simulink model "sm_car"  (R2022a)
settings: Solver=ode23t  StartTime=0.0  StopTime=200  MaxStep=0.4  RelTol=1e-3  AbsTol=1e-3  EnableMultiTasking=on
PreLoadFcn:
  | disp('Loading default data for 2-axle vehicle and 1-axle trailer.')
  | if verLessThan('matlab', '9.11')
  |     load Vehicle_139
  |     Vehicle = Vehicle_139;
  |     load Trailer_01
  |     Trailer = Trailer_01;
  | else
  |     load Vehicle_189
  |     Vehicle = Vehicle_189;
  |     load Trailer_07
  |     Trailer = Trailer_07;
  | end
  | 
  | disp('Turning off MFEval warnings...')
  | disp('Solver:CoeffChecks:Eyk -- OFF')
  | disp('Solver:Limits:Exceeded -- OFF')
  | disp('Solver:CoeffChecks:Et -- OFF')
  | disp('Solver:CoeffChecks:Exa -- OFF')
  | 
  | warning('off','Solver:CoeffChecks:Eyk')
  | warning('off','Solver:Limits:Exceeded')
  | warning('off','Solver:CoeffChecks:Et')
  | warning('off','Solver:CoeffChecks:Exa')
  | %warning('off','Solver:Radius:NegativeRho')
  | 
  | % Due to usability issue in Repeating Sequence block
  | warning('off','Simulink:Masking:Invalid');
  | 
  | % Eliminate unnecessary warnings in inactive variants
  | % Warnings generated only if you click through inactive variant
  | warning('off','MATLAB:nonExistentField');
  | warning('off','Simulink:Parameters:BlkParamUndefined');
PostLoadFcn:
  | disp('Disabling trailer by default.')
  | set_param([bdroot '/Vehicle'],'popup_trailer','Off')
  | warning('off','sm:sli:setup:compile:LocalSolverNotSupported')
  | sm_car_config_maneuver(bdroot,'WOT Braking');
  | sm_car_config_vehicle(bdroot);
  | sm_car_config_logging(bdroot);
InitFcn:
  | sm_car_config_camera;
  | Vehicle = sm_car_vehcfg_checkConfig(Vehicle);
  | sm_car_check_tire_model(bdroot);
  | addpath('C:\MasterThesis_CEVT\code\casadi-windows-matlabR2016a-v3.5.5')
  | addpath('C:\MasterThesis_CEVT\code')
  | addpath('C:\MasterThesis_CEVT\code\python scripts')
StartFcn:
  | tic;
StopFcn:
  | Elapsed_Sim_Time = toc;
  | % disp(['Elapsed Sim Time = ' num2str(Elapsed_Sim_Time)]);
  | % Run script that exports relevant simulation data to json
  | simToJson
undefined symbols (not defined in the file or in its folder): Control, Driver, Maneuver
libraries: sm_car_lib x22, simulink x17, sm_lib x3, Vehicle_Visualization x3, Driver_Long_Lat_Stanley x2, Maneuver_Get_Pose x2, Camera_Frame_Definitions x1, Control_FuelCell1Motor x1, slpidlib x1, Driver_Drive_Cycle x1, Driver_Gamepad_Xbox x1, Driver_Open_Loop x1
(part 3 of 3)

== system sm_car/Vehicle/Vehicle Constraint/No Yaw ==
  Cartesian Joint : sm_lib/Joints/Cartesian Joint  JointMode=Normal  SenseConstraintForce=off  SenseConstraintForceX=off  SenseConstraintForceY=off  SenseConstraintForceZ=off  SenseConstraintTorque=off  SenseConstraintTorqueX=off  SenseConstraintTorqueY=off  SenseConstraintTorqueZ=off  SenseTotalForce=off  SenseTotalForceX=off  SenseTotalForceY=off  SenseTotalForceZ=off  SenseTotalTorque=off  SenseTotalTorqueX=off  SenseTotalTorqueY=off  SenseTotalTorqueZ=off  CompositeWrenchDir=FollowerOnBase  CompositeWrenchFrame=BaseFrame  PxEquilibriumPosition=0  PxEquilibriumPositionUnits=m  PxSpringStiffness=0  PxSpringStiffnessUnits=N/m  PxDampingCoefficient=0  PxDampingCoefficientUnits=N/(m/s)  PxTorqueActuationMode=NoTorque  PxMotionActuationMode=ComputedMotion  PxSensePosition=off  PxSenseVelocity=off  PxSenseAcceleration=off  PxSenseTorqueForce=off  PxSenseLowerLimitTorqueForce=off  PxSenseUpperLimitTorqueForce=off  PxLowerLimitSpecify=off  PxLowerLimitBound=-1  PxLowerLimitBoundUnits=m  PxLowerLimitStiffness=1e6  PxLowerLimitStiffnessUnits=N/m  PxLowerLimitDamping=1e3  PxLowerLimitDampingUnits=N/(m/s)  PxLowerLimitTransitionRegionWidth=1e-4  PxLowerLimitTransitionRegionWidthUnits=m  PxUpperLimitSpecify=off  PxUpperLimitBound=1  PxUpperLimitBoundUnits=m  PxUpperLimitStiffness=1e6  PxUpperLimitStiffnessUnits=N/m  PxUpperLimitDamping=1e3  PxUpperLimitDampingUnits=N/(m/s)  PxUpperLimitTransitionRegionWidth=1e-4  PxUpperLimitTransitionRegionWidthUnits=m  PxPositionTargetSpecify=off  PxPositionTargetPriority=High  PxPositionTargetValue=0  PxPositionTargetValueUnits=m  PxVelocityTargetSpecify=off  PxVelocityTargetPriority=High  PxVelocityTargetValue=0  PxVelocityTargetValueUnits=m/s  PyEquilibriumPosition=0  PyEquilibriumPositionUnits=m  PySpringStiffness=0  PySpringStiffnessUnits=N/m  PyDampingCoefficient=0  PyDampingCoefficientUnits=N/(m/s)  PyTorqueActuationMode=NoTorque  PyMotionActuationMode=ComputedMotion  PySensePosition=off  PySenseVelocity=off  PySenseAcceleration=off  PySenseTorqueForce=off  PySenseLowerLimitTorqueForce=off  PySenseUpperLimitTorqueForce=off  PyLowerLimitSpecify=off  PyLowerLimitBound=-1  PyLowerLimitBoundUnits=m  PyLowerLimitStiffness=1e6  PyLowerLimitStiffnessUnits=N/m  PyLowerLimitDamping=1e3  PyLowerLimitDampingUnits=N/(m/s)  PyLowerLimitTransitionRegionWidth=1e-4  PyLowerLimitTransitionRegionWidthUnits=m  PyUpperLimitSpecify=off  PyUpperLimitBound=1  PyUpperLimitBoundUnits=m  PyUpperLimitStiffness=1e6  PyUpperLimitStiffnessUnits=N/m  PyUpperLimitDamping=1e3  PyUpperLimitDampingUnits=N/(m/s)  PyUpperLimitTransitionRegionWidth=1e-4  PyUpperLimitTransitionRegionWidthUnits=m  PyPositionTargetSpecify=off  PyPositionTargetPriority=High  PyPositionTargetValue=0  PyPositionTargetValueUnits=m  PyVelocityTargetSpecify=off  PyVelocityTargetPriority=High  PyVelocityTargetValue=0  PyVelocityTargetValueUnits=m/s  PzEquilibriumPosition=0  PzEquilibriumPositionUnits=m  PzSpringStiffness=0  PzSpringStiffnessUnits=N/m  PzDampingCoefficient=0  PzDampingCoefficientUnits=N/(m/s)  PzTorqueActuationMode=NoTorque  PzMotionActuationMode=ComputedMotion  PzSensePosition=off  PzSenseVelocity=off  PzSenseAcceleration=off  PzSenseTorqueForce=off  PzSenseLowerLimitTorqueForce=off  PzSenseUpperLimitTorqueForce=off  PzLowerLimitSpecify=off  PzLowerLimitBound=-1  PzLowerLimitBoundUnits=m  PzLowerLimitStiffness=1e6  PzLowerLimitStiffnessUnits=N/m  PzLowerLimitDamping=1e3  PzLowerLimitDampingUnits=N/(m/s)  PzLowerLimitTransitionRegionWidth=1e-4  PzLowerLimitTransitionRegionWidthUnits=m  PzUpperLimitSpecify=off  PzUpperLimitBound=1  PzUpperLimitBoundUnits=m  PzUpperLimitStiffness=1e6  PzUpperLimitStiffnessUnits=N/m  PzUpperLimitDamping=1e3  PzUpperLimitDampingUnits=N/(m/s)  PzUpperLimitTransitionRegionWidth=1e-4  PzUpperLimitTransitionRegionWidthUnits=m  PzPositionTargetSpecify=off  PzPositionTargetPriority=High  PzPositionTargetValue=0  PzPositionTargetValueUnits=m  PzVelocityTargetSpecify=off  PzVelocityTargetPriority=High  PzVelocityTargetValue=0  PzVelocityTargetValueUnits=m/s
  Universal Joint : sm_lib/Joints/Universal Joint  JointMode=Normal  SenseConstraintForce=off  SenseConstraintForceX=off  SenseConstraintForceY=off  SenseConstraintForceZ=off  SenseConstraintTorque=off  SenseConstraintTorqueX=off  SenseConstraintTorqueY=off  SenseConstraintTorqueZ=off  SenseTotalForce=off  SenseTotalForceX=off  SenseTotalForceY=off  SenseTotalForceZ=off  SenseTotalTorque=off  SenseTotalTorqueX=off  SenseTotalTorqueY=off  SenseTotalTorqueZ=off  CompositeWrenchDir=FollowerOnBase  CompositeWrenchFrame=BaseFrame  RxEquilibriumPosition=0  RxEquilibriumPositionUnits=deg  RxSpringStiffness=0  RxSpringStiffnessUnits=N*m/deg  RxDampingCoefficient=0  RxDampingCoefficientUnits=N*m/(deg/s)  RxTorqueActuationMode=NoTorque  RxMotionActuationMode=ComputedMotion  RxSensePosition=off  RxSenseVelocity=off  RxSenseAcceleration=off  RxSenseTorqueForce=off  RxSenseLowerLimitTorqueForce=off  RxSenseUpperLimitTorqueForce=off  RxLowerLimitSpecify=off  RxLowerLimitBound=-90  RxLowerLimitBoundUnits=deg  RxLowerLimitStiffness=1e4  RxLowerLimitStiffnessUnits=N*m/deg  RxLowerLimitDamping=10  RxLowerLimitDampingUnits=N*m/(deg/s)  RxLowerLimitTransitionRegionWidth=0.1  RxLowerLimitTransitionRegionWidthUnits=deg  RxUpperLimitSpecify=off  RxUpperLimitBound=90  RxUpperLimitBoundUnits=deg  RxUpperLimitStiffness=1e4  RxUpperLimitStiffnessUnits=N*m/deg  RxUpperLimitDamping=10  RxUpperLimitDampingUnits=N*m/(deg/s)  RxUpperLimitTransitionRegionWidth=0.1  RxUpperLimitTransitionRegionWidthUnits=deg  RxPositionTargetSpecify=off  RxPositionTargetPriority=High  RxPositionTargetValue=0  RxPositionTargetValueUnits=deg  RxVelocityTargetSpecify=off  RxVelocityTargetPriority=High  RxVelocityTargetValue=0  RxVelocityTargetValueUnits=deg/s  RyEquilibriumPosition=0  RyEquilibriumPositionUnits=deg  RySpringStiffness=0  RySpringStiffnessUnits=N*m/deg  RyDampingCoefficient=0  RyDampingCoefficientUnits=N*m/(deg/s)  RyTorqueActuationMode=NoTorque  RyMotionActuationMode=ComputedMotion  RySensePosition=off  RySenseVelocity=off  RySenseAcceleration=off  RySenseTorqueForce=off  RySenseLowerLimitTorqueForce=off  RySenseUpperLimitTorqueForce=off  RyLowerLimitSpecify=off  RyLowerLimitBound=-90  RyLowerLimitBoundUnits=deg  RyLowerLimitStiffness=1e4  RyLowerLimitStiffnessUnits=N*m/deg  RyLowerLimitDamping=10  RyLowerLimitDampingUnits=N*m/(deg/s)  RyLowerLimitTransitionRegionWidth=0.1  RyLowerLimitTransitionRegionWidthUnits=deg  RyUpperLimitSpecify=off  RyUpperLimitBound=90  RyUpperLimitBoundUnits=deg  RyUpperLimitStiffness=1e4  RyUpperLimitStiffnessUnits=N*m/deg  RyUpperLimitDamping=10  RyUpperLimitDampingUnits=N*m/(deg/s)  RyUpperLimitTransitionRegionWidth=0.1  RyUpperLimitTransitionRegionWidthUnits=deg  RyPositionTargetSpecify=off  RyPositionTargetPriority=High  RyPositionTargetValue=0  RyPositionTargetValueUnits=deg  RyVelocityTargetSpecify=off  RyVelocityTargetPriority=High  RyVelocityTargetValue=0  RyVelocityTargetValueUnits=deg/s
  F : PMIOPort  Side=Right
  B : PMIOPort  Port=2  Side=Left
  connections:
  Cartesian Joint/LConn1 -- B/RConn1
  Cartesian Joint/RConn1 -- Universal Joint/LConn1
  Universal Joint/RConn1 -- F/RConn1

== system sm_car/Visualization/Unreal/Animation Off ==
  xyz : Inport
  rpy : Inport  Port=2
  ws : Inport  Port=3
  aCamber : Inport  Port=4
  aSteerWheel : Inport  Port=5
  Terminator{,1..4} (5 alike) : Terminator
  wires:
  rpy/1 -> Terminator1/1
  aSteerWheel/1 -> Terminator4/1
  aCamber/1 -> Terminator3/1
  xyz/1 -> Terminator/1
  ws/1 -> Terminator2/1

== system sm_car/Visualization/Unreal/Animation On ==
  xyz : Inport
  rpy : Inport  Port=2
  ws : Inport  Port=3
  aCamber : Inport  Port=4
  aSteerWheel : Inport  Port=5
  Transform Data for Uneal : Vehicle_Visualization/Transform Data for Unreal  SystemSampleTime=-1  VariantActivationTime=update diagram  Latency=0  AutoFrameSizeCalculation=off
  Unreal Animation : Subsystem
  wires:
  Transform Data for Uneal/2 -> Unreal Animation/2(Rotation)  "Unreal_Rotation"
  Transform Data for Uneal/1 -> Unreal Animation/1(Translation)  "Unreal_Translation"
  ws/1 -> Transform Data for Uneal/3
  xyz/1 -> Transform Data for Uneal/1
  aCamber/1 -> Transform Data for Uneal/4
  aSteerWheel/1 -> Transform Data for Uneal/5
  rpy/1 -> Transform Data for Uneal/2

== system sm_car/Visualization/XY Plot/XY Plot Off ==
  VehBus : Inport
  DrvBus : Inport  Port=2
  Terminator : Terminator
  Terminator1 : Terminator
  wires:
  VehBus/1 -> Terminator/1
  DrvBus/1 -> Terminator1/1

== system sm_car/Controller/Battery 2 Motor/Regen Torque Limit/Check Within Limits ==
  up : Inport
  lo : Inport  Port=2
  u : Inport  Port=3
  Compare To Zero : simulink/Logic and Bit Operations/Compare To Zero  relop=>=  OutDataTypeStr=boolean
  Compare To Zero1 : simulink/Logic and Bit Operations/Compare To Zero  relop=<=  OutDataTypeStr=boolean
  Logical Operator : Logic  AllPortsSameDT=off  OutDataTypeStr=boolean
  Saturation Dynamic1 : simulink/Discontinuities/Saturation Dynamic  OutMin=[]  OutMax=[]  OutDataTypeStr=Inherit: Same as second input  OutDataType=fixdt(1, 16)  OutScaling=2^-10  DoSatur=off
  Subtract : Sum  Inputs=+-
  Subtract1 : Sum  Inputs=-+
  InLimit : Outport  SampleTime=0  VectorParamsAs1DForOutWhenUnconnected=off
  y : Outport  Port=2  VectorParamsAs1DForOutWhenUnconnected=off
  wires:
  Logical Operator/1 -> InLimit/1
  Compare To Zero1/1 -> Logical Operator/2
  Compare To Zero/1 -> Logical Operator/1
  Subtract1/1 -> Compare To Zero1/1
  Subtract/1 -> Compare To Zero/1
  u/1 -> Saturation Dynamic1/2, Subtract/2, Subtract1/1
  up/1 -> Saturation Dynamic1/1, Subtract/1
  lo/1 -> Saturation Dynamic1/3, Subtract1/2
  Saturation Dynamic1/1 -> y/1

== system sm_car/Controller/Battery 2 Motor/Regen Torque Limit/Mech to Elec Power Estimate ==
  note: Pelec_req = Pmech_req*Eff^k,
      | k = -1 if Motoring >= 0,
      | k = 1 if Generating < 0
  note: Using an Efficiency Map, we can estimate the
      | Electric Power from the Mechanical  Torque Request.
  note: Check if Motoring
      | or Generating
  MotTrqCmd : Inport
  MotSpd : Inport  Port=2
  Abs : Abs  ZeroCross=off  SaturateOnIntegerOverflow=off
  Abs1 : Abs  ZeroCross=off  SaturateOnIntegerOverflow=off
  Constant1 : Constant  Value=-1  SampleTime=0
  Constant2 : Constant  SampleTime=0
  Eff Map : Lookup_n-D  BreakpointsForDimension1=Control.MotorA1.LossTable.w.Value  BreakpointsForDimension2=Control.MotorA1.LossTable.trq.Value  Table=Control.MotorA1.LossTable.efficiency.Value  ExtrapMethod=Clip  UseLastTableValue=on  InternalRulePriority=Speed  OutDataTypeStr=Inherit: Inherit from 'Table data'  RndMeth=Simplest
      settings: InputPortMap=u0,u1
  Gain1 : Gain  Gain=1/100
  Math Function : Math  Operator=pow  SignedPower=on  OutputSignalType=real
  Product : Product
  Product3 : Product
  Product4 : Product
  Scope : Scope  NumInputPorts=4
  Switch2 : Switch  ZeroCross=off  SaturateOnIntegerOverflow=off  InputSameDT=off
  rads_to_rpm : Gain  Gain=30/pi
  MotPwrElecReq : Outport  VectorParamsAs1DForOutWhenUnconnected=off
  Eff2k : Outport  Port=2  VectorParamsAs1DForOutWhenUnconnected=off
  wires:
  MotTrqCmd/1 -> Abs1/1, Product/2, Scope/4, Product3/2
  MotSpd/1 -> rads_to_rpm/1, Scope/3, Product/1, Product3/1
  Product/1 -> Switch2/2
  rads_to_rpm/1 -> Abs/1
  Abs1/1 -> Eff Map/2
  Product4/1 -> Scope/2, MotPwrElecReq/1
  Math Function/1 -> Product4/2, Eff2k/1
  Gain1/1 -> Math Function/1
  Abs/1 -> Eff Map/1
  Eff Map/1 -> Scope/1, Gain1/1
  Constant2/1 -> Switch2/3
  Constant1/1 -> Switch2/1
  Switch2/1 -> Math Function/2
  Product3/1 -> Product4/1

== system sm_car/Controller/Battery 2 Motor/Regen Torque Limit/Torque Limit ==
  MotTrq : Inport
  MotSpd : Inport  Port=2
  Gain : Gain  Gain=-1
  MaxMotTrqVsSpd : Lookup_n-D  NumberOfTableDimensions=1  BreakpointsForDimension1=Control.MotorA1.TorqueSpd.w.Value  Table=Control.MotorA1.TorqueSpd.trq.Value  ExtrapMethod=Clip  UseLastTableValue=on  InternalRulePriority=Speed  OutDataTypeStr=Inherit: Inherit from 'Table data'  RndMeth=Simplest
  Saturation Dynamic : simulink/Discontinuities/Saturation Dynamic  OutMin=[]  OutMax=[]  OutDataTypeStr=Inherit: Same as second input  OutDataType=fixdt(1, 16)  OutScaling=2^-10  DoSatur=off
  rads_to_rpm : Gain  Gain=30/pi
  MotReqCmd : Outport  VectorParamsAs1DForOutWhenUnconnected=off
  wires:
  Saturation Dynamic/1 -> MotReqCmd/1
  Gain/1 -> Saturation Dynamic/3
  rads_to_rpm/1 -> MaxMotTrqVsSpd/1
  MaxMotTrqVsSpd/1 -> Saturation Dynamic/1, Gain/1
  MotSpd/1 -> rads_to_rpm/1
  MotTrq/1 -> Saturation Dynamic/2

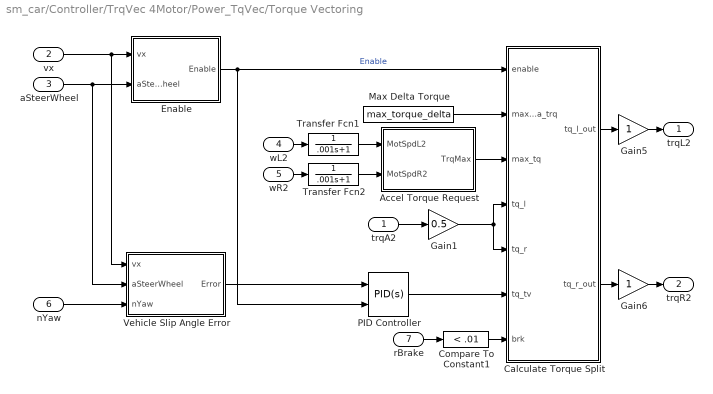
== system sm_car/Controller/TrqVec 4Motor/Power_TqVec/Torque Vectoring ==
  trqA2 : Inport
  vx : Inport  Port=2
  aSteerWheel : Inport  Port=3
  wL2 : Inport  Port=4
  wR2 : Inport  Port=5
  nYaw : Inport  Port=6
  rBrake : Inport  Port=7
  Accel Torque Request : Subsystem
  Calculate Torque Split : MATLAB Function  TreatAsAtomicUnit=on
  Compare To Constant1 : simulink/Logic and Bit Operations/Compare To Constant  relop=<  const=.01  OutDataTypeStr=boolean
  Enable : Subsystem
  Gain1 : Gain  Gain=0.5
  Gain5 : Gain
  Gain6 : Gain
  Max Delta Torque : Constant  Value=max_torque_delta
  PID Controller : slpidlib/PID Controller  Controller=PID  Form=Parallel  TimeDomain=Continuous-time  UseExternalTs=off  SampleTime=-1  IntegratorMethod=Forward Euler  FilterMethod=Forward Euler  ControllerParametersSource=internal  P=P  I=I  UseKiTs=off  D=0  N=1  UseFilter=on  TunerSelectOption=Transfer Function Based (PID Tuner App)  InitialConditionSource=internal  InitialConditionForIntegrator=0  InitialConditionForFilter=0  DifferentiatorICPrevScaledInput=0  ExternalReset=either  TrackingMode=off  Kt=1  LimitOutput=off  SatLimitsSource=internal  UpperSaturationLimit=inf  LowerSaturationLimit=-inf  LinearizeAsGain=on  AntiWindupMode=back-calculation  Kb=1  POutMin=[]  POutMax=[]  IOutMin=[]  IOutMax=[]  DOutMin=[]  DOutMax=[]  NOutMin=[]  NOutMax=[]  SumOutMin=[]  SumOutMax=[]  SaturationOutMin=[]  SaturationOutMax=[]  PParamMin=[]  PParamMax=[]  IParamMin=[]  IParamMax=[]  DParamMin=[]  DParamMax=[]  NParamMin=[]  NParamMax=[]  KbParamMin=[]  KbParamMax=[]  KtParamMin=[]  KtParamMax=[]  KbOutMin=[]  KbOutMax=[]  KtOutMin=[]  KtOutMax=[]  IntegratorOutMin=[]  IntegratorOutMax=[]  FilterOutMin=[]  FilterOutMax=[]  SumI1OutMin=[]  SumI1OutMax=[]  SumI2OutMin=[]  SumI2OutMax=[]  SumI3OutMin=[]  SumI3OutMax=[]  SumI4OutMin=[]  SumI4OutMax=[]  SumDOutMin=[]  SumDOutMax=[]  DifferentiatorOutMin=[]  DifferentiatorOutMax=[]  FilterDiffOutCoefMin=[]  FilterDiffOutCoefMax=[]  ReciprocalOutMin=[]  ReciprocalOutMax=[]  SumDenOutMin=[]  SumDenOutMax=[]  SumNumOutMin=[]  SumNumOutMax=[]  DivideOutMin=[]  DivideOutMax=[]  UdiffTsProdOutMin=[]  UdiffTsProdOutMax=[]  NTsProdOutMin=[]  NTsProdOutMax=[]  UintegralTsProdOutMin=[]  UintegralTsProdOutMax=[]  UngainTsProdOutMin=[]  UngainTsProdOutMax=[]  IntegratorContinuousStateAttributes=''  IntegratorStateMustResolveToSignalObject=off  IntegratorRTWStateStorageClass=Auto  FilterContinuousStateAttributes=''  FilterStateMustResolveToSignalObject=off  FilterRTWStateStorageClass=Auto  ParallelPVariant=InternalParameters  IdealPVariant=Disabled  IVariant=InternalParameters  DVariant=InternalParameters  IntegratorVariant=Continuous  SatVariant=Disabled  AWVariant=Passthrough  PCopyVariant=Disabled  TRVariant=Disabled  FdbkBlocksVariant=Forward  IdealPFdbkVariant=Disabled  SatFdbkVariant=Disabled  DerivativeFilterVariant=ContFilter  NVariant=InternalParameters  NCopyVariant=Disabled  FilterICVariant=InternalICsFilter  IntegratorICVariant=InternalICs  ExternalResetVariant=ExternalReset  TRSumVariant=Passthrough  SumFdbkVariant=Disabled  SumVariant=Sum_PID  TsampFilterVariant=InternalTs  TsampNgainVariant=Passthrough  TsampIntegralVariant=Passthrough  ExternalSaturationOutDataTypeStr=Inherit: Same as second input  aMode=0
  Transfer Fcn1 : TransferFcn  Denominator=[.001 1]
  Transfer Fcn2 : TransferFcn  Denominator=[.001 1]
  Vehicle Slip Angle Error : Subsystem
  trqL2 : Outport  VectorParamsAs1DForOutWhenUnconnected=off
  trqR2 : Outport  Port=2  VectorParamsAs1DForOutWhenUnconnected=off
  wires:
  wL2/1 -> Transfer Fcn1/1
  Transfer Fcn1/1 -> Accel Torque Request/1(MotSpdL2)
  Accel Torque Request/1(TrqMax) -> Calculate Torque Split/3(max_tq)
  vx/1 -> Vehicle Slip Angle Error/1(vx), Enable/1(vx)
  aSteerWheel/1 -> Vehicle Slip Angle Error/2(aSteerWheel), Enable/2(aSteerWheel)
  Gain5/1 -> trqL2/1
  PID Controller/1 -> Calculate Torque Split/6(tq_tv)
  wR2/1 -> Transfer Fcn2/1
  Calculate Torque Split/2(tq_r_out) -> Gain6/1
  trqA2/1 -> Gain1/1
  Transfer Fcn2/1 -> Accel Torque Request/2(MotSpdR2)
  Compare To Constant1/1 -> Calculate Torque Split/7(brk)
  Calculate Torque Split/1(tq_l_out) -> Gain5/1
  Vehicle Slip Angle Error/1(Error) -> PID Controller/1
  Gain6/1 -> trqR2/1
  rBrake/1 -> Compare To Constant1/1
  Gain1/1 -> Calculate Torque Split/5(tq_r), Calculate Torque Split/4(tq_l)
  Enable/1(Enable) -> PID Controller/2, Calculate Torque Split/1(enable)  "Enable"
  nYaw/1 -> Vehicle Slip Angle Error/3(nYaw)
  Max Delta Torque/1 -> Calculate Torque Split/2(max_delta_trq)

== system sm_car/Driver/Interactive/Pace Car/None ==
  "VehBus " : Inport
  Terminator : Terminator
  wires:
  "VehBus "/1 -> Terminator/1

== system sm_car/Driver/Interactive/Pace Car/Show ==
  "VehBus " : Inport
  Maneuver : Maneuver_Get_Pose/Maneuver  Maneuver=Maneuver  popup_window=No
  Terminator{,1..3} (4 alike) : Terminator
  wires:
  ? -> Terminator3/1
  Maneuver/3 -> Terminator2/1
  Maneuver/2 -> Terminator1/1
  Maneuver/1 -> Terminator/1
  "VehBus "/1 -> Maneuver/1

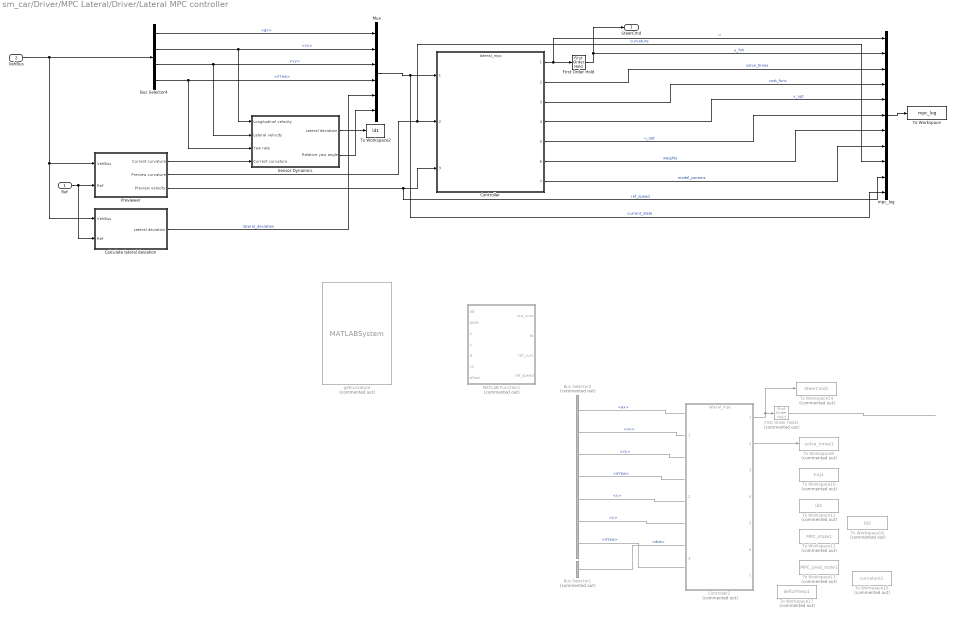
== system sm_car/Driver/MPC Lateral/Driver/Lateral MPC controller ==
  Ref : Inport
  VehBus : Inport  Port=2
  Bus Selector1 : BusSelector  Commented=on  OutputSignals=dist
  Bus Selector2 : BusSelector  Commented=on  OutputSignals=Chassis.Body.CG.ax,Chassis.Body.CG.vx,Chassis.Body.CG.vy,World.aYaw,World.x,World.y,World.nYaw
  Bus Selector4 : BusSelector  OutputSignals=Chassis.Body.CG.gx,Chassis.Body.CG.vx,Chassis.Body.CG.vy,World.nYaw
  Calculate lateral deviation : Subsystem
  Controller : ModelReference  ModelNameDialog=lateral_mpc.slx  SimulationMode=Normal  CachedPortDiscreteRates=[-1]  ModelReferenceVersion=4.57
  Controller1 : ModelReference  Commented=on  ModelNameDialog=lateral_mpc.slx  SimulationMode=Normal  CachedPortDiscreteRates=[-1]  ModelReferenceVersion=4.57
  First Order Hold : FirstOrderHold  ErrorTolerance=inf
  First Order Hold1 : FirstOrderHold  Commented=on  ErrorTolerance=inf
  MATLAB Function1 : MATLAB Function  Commented=on  SystemSampleTime=0.1
  Mux : Mux  Inputs=6
  Previewer : Subsystem
  Sensor Dynamics : Subsystem
  To Workspace : ToWorkspace  VariableName=mpc_log  SaveFormat=Timeseries  SampleTime=-1
  To Workspace10 : ToWorkspace  Commented=on  VariableName=traj1  SaveFormat=Structure With Time  SampleTime=-1
  To Workspace11 : ToWorkspace  Commented=on  VariableName=ld2  SaveFormat=Timeseries  SampleTime=-1
  To Workspace12 : ToWorkspace  Commented=on  VariableName=MPC_state1  SaveFormat=Timeseries  SampleTime=-1
  To Workspace13 : ToWorkspace  Commented=on  VariableName=MPC_pred_state1  SaveFormat=Timeseries  SampleTime=-1
  To Workspace14 : ToWorkspace  Commented=on  VariableName=SteerCmd1  SaveFormat=Timeseries  SampleTime=-1
  To Workspace15 : ToWorkspace  Commented=on  VariableName=curvature1  SaveFormat=Timeseries  SampleTime=-1
  To Workspace16 : ToWorkspace  Commented=on  VariableName=ld3  SaveFormat=Timeseries  SampleTime=-1
  To Workspace17 : ToWorkspace  Commented=on  VariableName=deltaTheta1  SaveFormat=Timeseries  SampleTime=-1
  To Workspace2 : ToWorkspace  VariableName=ld1  SaveFormat=Timeseries  SampleTime=-1
  To Workspace9 : ToWorkspace  Commented=on  VariableName=solve_times1  SaveFormat=Timeseries  SampleTime=-1
  getCurvature : MATLABSystem  Commented=on  System=getCurvature  x=Maneuver.Trajectory.x.Value  y=Maneuver.Trajectory.y.Value  N=50  Ts=0.1  d=Maneuver.Trajectory.xTrajectory.Value  vx=Maneuver.Trajectory.vx.Value  aYaw=Maneuver.Trajectory.aYaw.Value  SimulateUsing=Interpreted execution
      mask Type: getCurvature
      mask Display:
      | disp('getCurvature');
      | port_label('input',1,'pose');
      | port_label('input',2,'pd');
      | port_label('output',1,'cur_curv');
      | port_label('output',2,'ld');
      | port_label('output',3,'ref_curv');
  mpc_log : BusCreator  Inputs=11
  SteerCmd : Outport
  wires:
  ? -> To Workspace13/1
  Bus Selector2/7 -> ?  "<nYaw>"
  Bus Selector2/4 -> ?  "<aYaw>"
  ? -> To Workspace17/1
  Controller1/2 -> To Workspace9/1
  ? -> Bus Selector1/1
  ? -> To Workspace16/1
  Controller1/1 -> To Workspace14/1, First Order Hold1/1
  ? -> To Workspace15/1
  Bus Selector2/6 -> ?  "<y>"
  Bus Selector1/1 -> ?  "<dist>"
  ? -> To Workspace12/1
  Bus Selector2/5 -> ?  "<x>"
  ? -> To Workspace10/1
  Bus Selector2/3 -> ?  "<vy>"
  ? -> To Workspace11/1
  Bus Selector2/2 -> ?  "<vx>"
  First Order Hold1/1 -> ?
  Bus Selector2/1 -> ?  "<ax>"
  Mux/1 -> mpc_log/11, Controller/1  "current_state"
  Sensor Dynamics/2(Relative yaw angle) -> Mux/6
  Bus Selector4/2 -> Sensor Dynamics/1(Longitudinal velocity), Mux/2  "<vx>"
  Bus Selector4/3 -> Sensor Dynamics/2(Lateral velocity), Mux/3  "<vy>"
  Bus Selector4/4 -> Sensor Dynamics/3(Yaw rate), Mux/4  "<nYaw>"
  Controller/1 -> First Order Hold/1, mpc_log/1  "u"
  First Order Hold/1 -> SteerCmd/1, mpc_log/2  "u_foh"
  Previewer/1(Current curvature) -> Sensor Dynamics/4(Current curvature)
  Calculate lateral deviation/1(Lateral deviation) -> Mux/5  "lateral_deviation"
  Previewer/2(Preview curvature) -> mpc_log/9, Controller/2  "curvature"
  Previewer/3(Preview velocity) -> mpc_log/10, Controller/3  "ref_speed"
  Bus Selector4/1 -> Mux/1  "<gx>"
  Ref/1 -> Calculate lateral deviation/2(Ref), Previewer/2(Ref)
  VehBus/1 -> Bus Selector4/1, Calculate lateral deviation/1(VehBus), Previewer/1(VehBus)
  Controller/3 -> mpc_log/4  "cost_func"
  Sensor Dynamics/1(Lateral deviation) -> To Workspace2/1
  Controller/2 -> mpc_log/3  "solve_times"
  Controller/4 -> mpc_log/5  "x_opt"
  Controller/5 -> mpc_log/6  "u_opt"
  mpc_log/1 -> To Workspace/1
  Controller/6 -> mpc_log/7  "weights"
  Controller/7 -> mpc_log/8  "model_params"

== system sm_car/Driver/MPC Lateral/Maneuver/vx override ==
  note: Override speed signal using
      | gain (to set to zero) and/or with an
      | offset (for passing maneuver).
  vx : Inport
  Bus Selector2 : BusSelector  OutputSignals=offset,gain
  Constant5 : Constant  Value=Maneuver.Trajectory.vx.Value
  Product : Product
  Sum : Sum  Inputs=++|
  vx_ovr : Outport  VectorParamsAs1DForOutWhenUnconnected=off
  wires:
  vx/1 -> Bus Selector2/1
  Bus Selector2/2 -> Product/1  "<gain>"
  Sum/1 -> vx_ovr/1
  Constant5/1 -> Product/2
  Product/1 -> Sum/2
  Bus Selector2/1 -> Sum/1  "<offset>"

== system sm_car/Driver/MPC Lateral/Maneuver/x override ==
  note: Override speed signal using
      | gain (to set to zero) and/or with an
      | offset (for passing maneuver).
  x : Inport
  Bus Selector2 : BusSelector  OutputSignals=offset,gain
  Constant3 : Constant  Value=Maneuver.Trajectory.x.Value
  Product : Product
  Sum : Sum  Inputs=++|
  x_ovr : Outport  VectorParamsAs1DForOutWhenUnconnected=off
  wires:
  Bus Selector2/1 -> Sum/1  "<offset>"
  Product/1 -> Sum/2
  Constant3/1 -> Product/2
  Sum/1 -> x_ovr/1
  Bus Selector2/2 -> Product/1  "<gain>"
  x/1 -> Bus Selector2/1

== system sm_car/Driver/MPC Lateral/Maneuver/y override ==
  note: Override speed signal using
      | gain (to set to zero) and/or with an
      | offset (for passing maneuver).
  y : Inport
  Bus Selector2 : BusSelector  OutputSignals=offset,gain
  Constant4 : Constant  Value=Maneuver.Trajectory.y.Value
  Product : Product
  Sum : Sum  Inputs=++|
  y_ovr : Outport  VectorParamsAs1DForOutWhenUnconnected=off
  wires:
  y/1 -> Bus Selector2/1
  Bus Selector2/2 -> Product/1  "<gain>"
  Sum/1 -> y_ovr/1
  Constant4/1 -> Product/2
  Product/1 -> Sum/2
  Bus Selector2/1 -> Sum/1  "<offset>"

== system sm_car/Driver/MPC Lateral/Maneuver/z override ==
  note: Override speed signal using
      | gain (to set to zero) and/or with an
      | offset (for passing maneuver).
  z : Inport
  Bus Selector2 : BusSelector  OutputSignals=offset,gain
  Constant1 : Constant  Value=Maneuver.Trajectory.z.Value
  Product : Product
  Sum : Sum  Inputs=++|
  z_ovr : Outport  VectorParamsAs1DForOutWhenUnconnected=off
  wires:
  Bus Selector2/1 -> Sum/1  "<offset>"
  Product/1 -> Sum/2
  Constant1/1 -> Product/2
  Sum/1 -> z_ovr/1
  Bus Selector2/2 -> Product/1  "<gain>"
  z/1 -> Bus Selector2/1

== system sm_car/Visualization/Unreal/Animation On/Unreal Animation ==
  Translation : Inport  OutDataTypeStr=single  PortDimensions=[5,3]
  Rotation : Inport  Port=2  OutDataTypeStr=single  PortDimensions=[5,3]
  Rate Transition1 : RateTransition  Deterministic=off  OutPortSampleTime=0.03
  Rate Transition2 : RateTransition  Deterministic=off  OutPortSampleTime=0.03
  Scale : Subsystem
  Simulation 3D Scene Configuration : sim3dlib/Simulation 3D Scene Configuration  Priority=0  ProjectFormat=Default Scenes  SceneDesc=Double lane change  ProjectName=C:\Program Files\MATLAB\R2022a\toolbox\shared\sim3d_projects\automotive_project\UE4\WindowsNoEditor\VehicleSimulation.exe  ScenePath=/Game/Maps/HwStrght  vehTagList={'Scene Origin';'SimulinkVehicle1'}  vehTag=SimulinkVehicle1  OpVisEn=off  Ts=.03  EnableWindow=on  EnableRemoteAccess=off  EnableWeather=off  SunAltitude=40.0  SunAzimuth=90  clouds=10  wind=1  fog=0  rain=0  sensorTag=MainCamera1  sensorId=1  sensorName=MainCamera1  mountLoc=Origin  offsetFlag=off  tmountOffset=[0, 0, 0]  rmountOffset=[0, 0, 0]  HorizontalResolution=1280  VerticalResolution=720  HorizontalFOV=60  mountPoint=[0 0 0]  mountOrientation=[0 0 0]  aMode=aMode  ID=1
      settings: SourceProductBaseCode=VE,AE,DR,UV,VE
  Simulation 3D Vehicle : sim3dautolib/Simulation 3D Vehicle  Priority=-1  PassVehMesh=Sedan  MeshPath=/MathWorksSimulation/Vehicles/Muscle/Meshes/SK_MuscleCar.SK_MuscleCar  VehColor=Blue  ActorName=SimulinkVehicle1  VehLightsControl=off  HeadlightColor=[ 1, 1, 1 ]  HighBeamIntensity=100000  LowBeamIntensity=60000  HighBeamConeAngle=1.22  LowBeamConeAngle=1.22  LeftHeadlightOrientation=[ 0, 0 ]  RightHeadlightOrientation=[ 0, 0 ]  BrakelightIntensity=500  ReverselightIntensity=500  SignallightIntensity=500  SignallightPeriod=1  SignalPulseWidth=50  Translation=[0 0 1; 0 0 0; 0 0 0; 0 0 0; 0 0 0]  Rotation=[0 0 0; 0 0 0; 0 0 0; 0 0 0; 0 0 0]  Scale=ones( 5, 3 )  SampleTime=.03  ActorType=SimulinkVehicle  ID=1  aMode=2  ActorTag=SimulinkVehicle1
      settings: SourceProductBaseCode=VE,AE,DR,UV,VE
  wires:
  Rotation/1 -> Rate Transition2/1
  Rate Transition1/1 -> Simulation 3D Vehicle/1
  Translation/1 -> Rate Transition1/1
  Rate Transition2/1 -> Simulation 3D Vehicle/2
  Scale/1(ScaleOut) -> Simulation 3D Vehicle/3

== system sm_car/Controller/TrqVec 4Motor/Power_TqVec/Torque Vectoring/Accel Torque Request ==
  MotSpdL2 : Inport
  MotSpdR2 : Inport  Port=2
  MaxMotTrqVsSpdA1 : Lookup_n-D  NumberOfTableDimensions=1  BreakpointsForDimension1=Control.MotorR2.TorqueSpd.w.Value  Table=Control.MotorL2.TorqueSpd.trq.Value  ExtrapMethod=Clip  UseLastTableValue=on  InternalRulePriority=Speed  OutDataTypeStr=Inherit: Inherit from 'Table data'  RndMeth=Simplest
  Terminator : Terminator
  rads_to_rpm : Gain  Gain=30/pi
  rads_to_rpm1 : Gain  Gain=30/pi
  TrqMax : Outport  VectorParamsAs1DForOutWhenUnconnected=off
  wires:
  rads_to_rpm/1 -> MaxMotTrqVsSpdA1/1
  MotSpdL2/1 -> rads_to_rpm/1
  MaxMotTrqVsSpdA1/1 -> TrqMax/1
  MotSpdR2/1 -> rads_to_rpm1/1
  rads_to_rpm1/1 -> Terminator/1

== system sm_car/Controller/TrqVec 4Motor/Power_TqVec/Torque Vectoring/Enable ==
  vx : Inport
  aSteerWheel : Inport  Port=2
  Abs : Abs  ZeroCross=off  SaturateOnIntegerOverflow=off
  Enable aSteerWheel : simulink/Logic and Bit Operations/Compare To Constant  relop=>  const=aSteerWheel_enable  OutDataTypeStr=boolean  ZeroCross=off
  Enable vx : simulink/Logic and Bit Operations/Compare To Constant  relop=>  const=vx_enable  OutDataTypeStr=boolean  ZeroCross=off
  Logical Operator : Logic  AllPortsSameDT=off  OutDataTypeStr=boolean
  Scope : Scope  NumInputPorts=3
  Enable : Outport  VectorParamsAs1DForOutWhenUnconnected=off
  wires:
  Enable aSteerWheel/1 -> Logical Operator/2
  Enable vx/1 -> Logical Operator/1
  Logical Operator/1 -> Scope/3, Enable/1
  vx/1 -> Enable vx/1, Scope/1
  aSteerWheel/1 -> Abs/1
  Abs/1 -> Enable aSteerWheel/1, Scope/2

== system sm_car/Controller/TrqVec 4Motor/Power_TqVec/Torque Vectoring/Vehicle Slip Angle Error ==
  vx : Inport
  aSteerWheel : Inport  Port=2
  nYaw : Inport  Port=3
  Add1 : Sum  Inputs=-+
  Distance Yaw Ctr Front Axle : Constant  Value=Vehicle.Chassis.Body.sAxle2.Value(1)/(-2)
  Divide3 : Product  Inputs=*/
  Multiply2 : Product
  Mux : Mux  Inputs=2
  Scope : Scope  NumInputPorts=2
  Steering Wheel to Driving Wheel : Gain  Gain=aStr_to_aWhl
  Error : Outport  VectorParamsAs1DForOutWhenUnconnected=off
  wires:
  Divide3/1 -> Mux/1, Add1/1  "Vehicle Slip Angle"
  vx/1 -> Divide3/2
  Add1/1 -> Error/1, Scope/2  "Error"
  nYaw/1 -> Multiply2/2
  aSteerWheel/1 -> Steering Wheel to Driving Wheel/1
  Distance Yaw Ctr Front Axle/1 -> Multiply2/1
  Steering Wheel to Driving Wheel/1 -> Add1/2, Mux/2  "Wheel Angle"
  Multiply2/1 -> Divide3/1
  Mux/1 -> Scope/1

== system sm_car/Driver/MPC Lateral/Driver/Lateral MPC controller/Calculate lateral deviation ==
  VehBus : Inport
  Ref : Inport  Port=2
  Bus Selector : BusSelector  OutputSignals=dist
  Bus Selector4 : BusSelector  OutputSignals=World.x,World.y,World.aYaw
  MATLAB Function2 : MATLAB Function  TreatAsAtomicUnit=on
  Mux1 : Mux  Inputs=3
  Mux2 : Mux  Inputs=3
  theta : Lookup_n-D  NumberOfTableDimensions=1  BreakpointsForDimension1=Maneuver.Trajectory.xTrajectory.Value  Table=Maneuver.Trajectory.aYaw.Value  InternalRulePriority=Speed  RndMeth=Simplest
  wrap angle : MATLAB Function  TreatAsAtomicUnit=on
  x : Lookup_n-D  NumberOfTableDimensions=1  BreakpointsForDimension1=Maneuver.Trajectory.xTrajectory.Value  Table=Maneuver.Trajectory.x.Value  InternalRulePriority=Speed  RndMeth=Simplest
  y : Lookup_n-D  NumberOfTableDimensions=1  BreakpointsForDimension1=Maneuver.Trajectory.xTrajectory.Value  Table=Maneuver.Trajectory.y.Value  InternalRulePriority=Speed  RndMeth=Simplest
  Lateral deviation : Outport
  wires:
  Mux2/1 -> MATLAB Function2/2(refPose)  "refPose"
  Mux1/1 -> MATLAB Function2/1(curPose)
  x/1 -> Mux2/1
  y/1 -> Mux2/2
  wrap angle/1(aYaw) -> Mux1/3
  VehBus/1 -> Bus Selector4/1
  Bus Selector4/3 -> wrap angle/1(u)  "<aYaw>"
  Bus Selector4/2 -> Mux1/2  "<y>"
  Bus Selector4/1 -> Mux1/1  "<x>"
  Ref/1 -> Bus Selector/1
  MATLAB Function2/1(ld) -> Lateral deviation/1
  Bus Selector/1 -> theta/1, x/1, y/1  "<dist>"
  theta/1 -> Mux2/3

== system sm_car/Driver/MPC Lateral/Driver/Lateral MPC controller/Previewer ==
  VehBus : Inport
  Ref : Inport  Port=2
  1-D Lookup Table : Lookup_n-D  NumberOfTableDimensions=1  BreakpointsForDimension1=Maneuver.Trajectory.xTrajectory.Value  TableSource=Input port  Table=tanh([-5:5])  InternalRulePriority=Speed  RndMeth=Simplest
      settings: InputPortMap=u0,p221
  1-D Lookup Table1 : Lookup_n-D  NumberOfTableDimensions=1  BreakpointsForDimension1=Maneuver.Trajectory.xTrajectory.Value  TableSource=Input port  Table=tanh([-5:5])  InternalRulePriority=Speed  RndMeth=Simplest
      settings: InputPortMap=u0,p221
  Bus Selector : BusSelector  OutputSignals=dist
  Bus Selector4 : BusSelector  OutputSignals=Chassis.Body.CG.vx
  Distance ref : Constant  Value=Maneuver.Trajectory.xTrajectory.Value
  Memory : Memory  InitialCondition=1
  To Workspace : ToWorkspace  VariableName=distance_along_traj  SaveFormat=Timeseries  SampleTime=-1
  Trajectory curvature : Subsystem  TreatAsAtomicUnit=on
  previewDist&Vel : MATLAB Function  TreatAsAtomicUnit=on  SystemSampleTime=0.1
      settings: RTWFcnNameOpts=Use subsystem name  RTWFileNameOpts=Use subsystem name
  v ref : Constant  Value=Maneuver.Trajectory.vx.Value
  Current curvature : Outport
  Preview curvature : Outport  Port=2
  Preview velocity : Outport  Port=3
  wires:
  Trajectory curvature/1(" ") -> Memory/1
  Trajectory curvature/2(curvature) -> 1-D Lookup Table1/2, 1-D Lookup Table/2
  Memory/1 -> Trajectory curvature/Enable
  v ref/1 -> previewDist&Vel/3(v_ref)
  Distance ref/1 -> previewDist&Vel/2(d_ref)
  previewDist&Vel/2(previewDist) -> 1-D Lookup Table/1
  previewDist&Vel/1(previewVel) -> Preview velocity/1
  Ref/1 -> Bus Selector/1
  1-D Lookup Table/1 -> Preview curvature/1
  1-D Lookup Table1/1 -> Current curvature/1
  Bus Selector/1 -> To Workspace/1, 1-D Lookup Table1/1, previewDist&Vel/1(ad)  "<dist>"
  Bus Selector4/1 -> previewDist&Vel/4(v0)  "<vx>"
  VehBus/1 -> Bus Selector4/1

== system sm_car/Driver/MPC Lateral/Driver/Lateral MPC controller/Sensor Dynamics ==
  Longitudinal velocity : Inport
  Lateral velocity : Inport  Port=2
  Yaw rate : Inport  Port=3
  Current curvature : Inport  Port=4
  Integrator : Integrator
  Integrator1 : Integrator
  Mux1 : Mux  Inputs=[1 1 1]
  Product : Product
  Subtract : Sum  Inputs=-+
  e1dot : Fcn  Expr=u(1)*u(3)+u(2)
  Lateral deviation : Outport  VectorParamsAs1DForOutWhenUnconnected=off
  Relative yaw angle : Outport  Port=2  VectorParamsAs1DForOutWhenUnconnected=off
  wires:
  Current curvature/1 -> Product/2
  Mux1/1 -> e1dot/1
  e1dot/1 -> Integrator1/1
  Longitudinal velocity/1 -> Mux1/1, Product/1
  Lateral velocity/1 -> Mux1/2
  Product/1 -> Subtract/1  "reference angular velocity"
  Integrator/1 -> Mux1/3, Relative yaw angle/1  "relative yaw angle"
  Yaw rate/1 -> Subtract/2
  Subtract/1 -> Integrator/1
  Integrator1/1 -> Lateral deviation/1  "lateral deviation"

== system sm_car/Visualization/Unreal/Animation On/Unreal Animation/Scale ==
  Constant{1..12,17,32..33} (15 alike) : Constant  OutDataTypeStr=single
  PartConcatenation : Subsystem
  ScaleOut : Outport  VectorParamsAs1DForOutWhenUnconnected=off
  wires:
  Constant10/1 -> PartConcatenation/15(WheelRearRightZ)
  Constant9/1 -> PartConcatenation/14(WheelRearRightY)
  Constant11/1 -> PartConcatenation/13(WheelRearRightX)
  Constant7/1 -> PartConcatenation/12(WheelRearLeftZ)
  Constant6/1 -> PartConcatenation/11(WheelRearLeftY)
  Constant8/1 -> PartConcatenation/10(WheelRearLeftX)
  Constant4/1 -> PartConcatenation/9(WheelFrontRightZ)
  Constant3/1 -> PartConcatenation/8(WheelFrontRightY)
  Constant5/1 -> PartConcatenation/7(WheelFrontRightX)
  Constant2/1 -> PartConcatenation/6(WheelFrontLeftZ)
  Constant1/1 -> PartConcatenation/5(WheelFrontLeftY)
  Constant33/1 -> PartConcatenation/4(WheelFrontLeftX)
  Constant32/1 -> PartConcatenation/3(BodyZ)
  Constant17/1 -> PartConcatenation/2(BodyY)
  Constant12/1 -> PartConcatenation/1(BodyX)
  PartConcatenation/1(ConcatOut) -> ScaleOut/1

== system sm_car/Driver/MPC Lateral/Driver/Lateral MPC controller/Previewer/Trajectory curvature ==
  Enable : EnablePort
  Constant : Constant  Value=Maneuver.Trajectory.x.Value
  Constant1 : Constant  Value=Maneuver.Trajectory.y.Value
  Constant2 : Constant  Value=0
  getCurvature : MATLAB Function  TreatAsAtomicUnit=on  SystemSampleTime=0.1
      settings: MinAlgLoopOccurrences=on  RTWFcnNameOpts=Use subsystem name  RTWFileNameOpts=Use subsystem name
  " " : Outport  InitialOutput=1
  curvature : Outport  Port=2
  wires:
  Constant/1 -> getCurvature/1(x)
  Constant1/1 -> getCurvature/2(y)
  getCurvature/1(curvature) -> curvature/1
  Constant2/1 -> " "/1

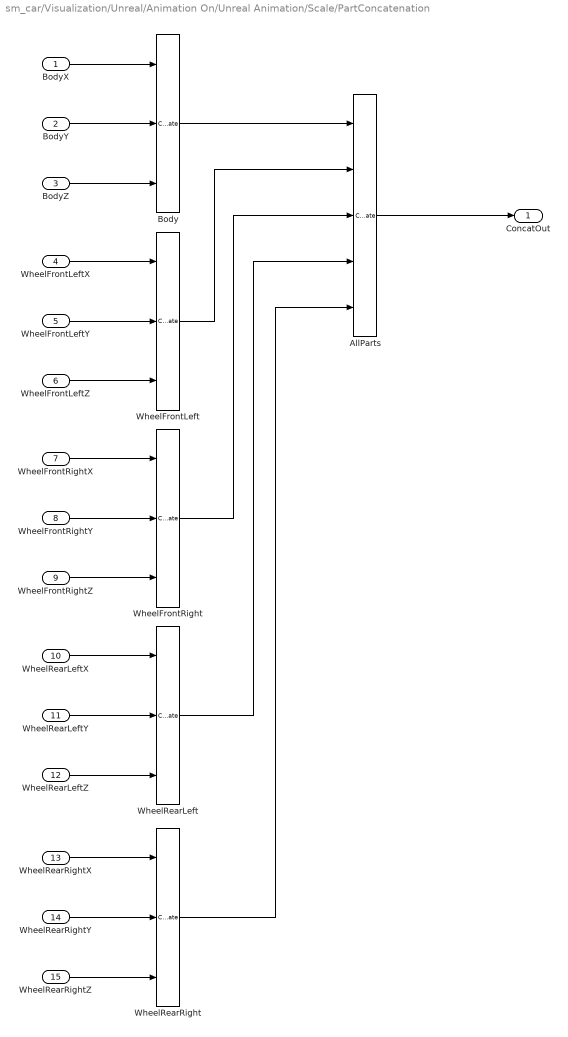
== system sm_car/Visualization/Unreal/Animation On/Unreal Animation/Scale/PartConcatenation ==
  BodyX : Inport
  BodyY : Inport  Port=2
  BodyZ : Inport  Port=3
  WheelFrontLeftX : Inport  Port=4
  WheelFrontLeftY : Inport  Port=5
  WheelFrontLeftZ : Inport  Port=6
  WheelFrontRightX : Inport  Port=7
  WheelFrontRightY : Inport  Port=8
  WheelFrontRightZ : Inport  Port=9
  WheelRearLeftX : Inport  Port=10
  WheelRearLeftY : Inport  Port=11
  WheelRearLeftZ : Inport  Port=12
  WheelRearRightX : Inport  Port=13
  WheelRearRightY : Inport  Port=14
  WheelRearRightZ : Inport  Port=15
  AllParts : Concatenate  NumInputs=5  Mode=Multidimensional array
  Body : Concatenate  NumInputs=3  Mode=Multidimensional array  ConcatenateDimension=2
  WheelFrontLeft : Concatenate  NumInputs=3  Mode=Multidimensional array  ConcatenateDimension=2
  WheelFrontRight : Concatenate  NumInputs=3  Mode=Multidimensional array  ConcatenateDimension=2
  WheelRearLeft : Concatenate  NumInputs=3  Mode=Multidimensional array  ConcatenateDimension=2
  WheelRearRight : Concatenate  NumInputs=3  Mode=Multidimensional array  ConcatenateDimension=2
  ConcatOut : Outport  VectorParamsAs1DForOutWhenUnconnected=off
  wires:
  BodyX/1 -> Body/1
  BodyZ/1 -> Body/3
  WheelFrontLeftX/1 -> WheelFrontLeft/1
  WheelFrontLeftZ/1 -> WheelFrontLeft/3
  WheelFrontLeftY/1 -> WheelFrontLeft/2
  BodyY/1 -> Body/2
  WheelFrontLeft/1 -> AllParts/2
  WheelRearRightX/1 -> WheelRearRight/1
  Body/1 -> AllParts/1
  WheelRearLeft/1 -> AllParts/4
  WheelFrontRight/1 -> AllParts/3
  WheelRearRightZ/1 -> WheelRearRight/3
  WheelFrontRightY/1 -> WheelFrontRight/2
  WheelFrontRightX/1 -> WheelFrontRight/1
  WheelRearRightY/1 -> WheelRearRight/2
  WheelRearLeftZ/1 -> WheelRearLeft/3
  AllParts/1 -> ConcatOut/1
  WheelRearLeftY/1 -> WheelRearLeft/2
  WheelRearRight/1 -> AllParts/5
  WheelRearLeftX/1 -> WheelRearLeft/1
  WheelFrontRightZ/1 -> WheelFrontRight/3

== matlab function sm_car/Driver/MPC Lateral/Driver/Lateral MPC controller/MATLAB Function1 ==
  data: cur_curv output; ad input; pose input; ld output; ref_curv output; ref_speed output; x input; y input; d input; vx input; aYaw input
function [cur_curv, ld, ref_curv, ref_speed] = getCurvature(ad, pose, x, y, d, vx, aYaw)
            N = 50;
            Ts = 0.1;
            ref_speed = zeros(1, N);
            ref_dist = zeros(1, N);
            ref_dist(1) = ad;
            for i = 1:N
                ref_speed(i) = interp1(d, vx, ref_dist(i), 'pchip');
                ref_dist(i+1) = ref_dist(i) + Ts * ref_speed(i);
            end
%             traj = interp1(d, path, ref_dist,'pchip');       
            ref_curv = interp1(d, curvature, ref_dist(1:end-1),'linear');
            cur_curv = ref_curv(1);
            
            refX = interp1(d, path(:,1), ad);
            refY = interp1(d, path(:,2), ad);
            refTheta = interp1(d, aYaw, ad);
      
            dx = pose(1) - refX;
            dy = pose(2) - refY;
        
            refCosTheta = cos(refTheta);
            refSinTheta = sin(refTheta);
        
            % Normal at the root point
            refNormal = refCosTheta .* dy - refSinTheta .* dx;
        
            % Compute lateral deviation
            ld = vecnorm([dx, dy]')' .* sign(refNormal);

== matlab function sm_car/Driver/MPC Lateral/Driver/Lateral MPC controller/Previewer/previewDist&Vel ==
  data: previewVel output; previewDist output; ad input; d_ref input; v_ref input; v0 input
function [previewVel, previewDist] = preview_d_v(ad, d_ref, v_ref, v0)
            N = 50;
            Ts = 0.1;
            previewDist = zeros(1, N);
            previewVel = zeros(1, N);
            % Current distance
%             previewDist(1) = ad;
            % Use current velocity to get first preview distance
            previewDist(1) = ad + Ts * v0;
            % Use first preview of distance to get vel preview
            previewVel(1) = interp1(d_ref, v_ref, previewDist(1), 'pchip');
            for k = 1:N-1
                previewDist(k+1) = previewDist(k) + Ts * previewVel(k);
                previewVel(k+1) = interp1(d_ref, v_ref, previewDist(k+1), 'pchip');
            end

== matlab function sm_car/Driver/MPC Lateral/Driver/Lateral MPC controller/Calculate lateral deviation/MATLAB Function2 ==
  data: curPose input; ld output; refPose input
function ld = getLateralDeviation(curPose, refPose)

dx = curPose(1) - refPose(1);
dy = curPose(2) - refPose(2);

refCosTheta = cos(refPose(3));
refSinTheta = sin(refPose(3));

% Normal at the root point
refNormal = refCosTheta .* dy - refSinTheta .* dx;

% Compute lateral deviation
ld = vecnorm([dx, dy]')' .* sign(refNormal);

== matlab function sm_car/Driver/MPC Lateral/Driver/Lateral MPC controller/Previewer/Trajectory curvature/getCurvature ==
  data: curvature output; x input; y input
function curvature = getCurvature(x, y)
            DX = gradient(x);
            DY = gradient(y);
            D2Y = gradient(DY);
            D2X = gradient(DX);
            curvature = (DX.*D2Y - DY.*D2X) ./ (DX.^2 + DY.^2).^(3/2);

== matlab function sm_car/Controller/TrqVec 4Motor/Power_TqVec/Torque Vectoring/Calculate Torque Split ==
  data: enable input; max_delta_trq input; max_tq input; tq_l_out output; tq_l input; tq_r input; tq_r_out output; tq_tv input; brk input
function [tq_l_out,tq_r_out] = fcn(enable,max_delta_trq,max_tq,tq_l,tq_r,tq_tv,brk)

% enable: flag to turn on torque vectoring
%         True if steering wheel is turned and non-zero vehicle speed
% brk   : flag to turn on torque vectoring
%         True if not braking


% Limit difference in torque between tires lower of 
% (input parameter) and max/min motor torque
t_lim=min(max_tq-abs(tq_l),max_tq-abs(tq_r));
delta_t=min(max_delta_trq,min(t_lim,abs(tq_tv)))*sign(tq_tv)*enable;

if brk>0 
    % Not braking. Use torque vectoring
    tq_l_out=(tq_l-delta_t);
    tq_r_out=(tq_r+delta_t);
else
    % No adjustments due to torque vectoring
    tq_l_out=tq_l;
    tq_r_out=tq_r;
end

== matlab function sm_car/Driver/MPC Lateral/Driver/Lateral MPC controller/Calculate lateral deviation/wrap angle ==
  data: u input; aYaw output
function aYaw = fcn(u)

aYaw = robotics.internal.wrapToPi(u);

== matlab function sm_car/Driver/MPC Lateral/Maneuver/MATLAB Function ==
  data: ad output; vTarget output; p input; q input; posx input; posy input; posz input; xywin input; speed input; yaw input; dist input; pd input; maxld input; minSpd input; speedGain input; pd output; idx_ptMin output; idx_ptMin_prev input; ref_ayaw output
function [ad,vTarget,pd,idx_ptMin,ref_ayaw] = getPoseCurRef(p,q,posx,posy,posz,xywin,speed,yaw,dist,pd, maxld, minSpd, speedGain, idx_ptMin_prev)
% speed = speed*0+10;
npts = length(posx);

% Look for nearest point in a window near last evaluation
% Obtain window
if (idx_ptMin_prev == -1)
    % For first evaluation, use entire list of points
    ptlist = 1:npts;
elseif((idx_ptMin_prev-xywin)<1)
    % Window overlaps at lower end: take points from upper end
    win2 = (npts+idx_ptMin_prev-xywin):1:npts;
    win1 = 1:(idx_ptMin_prev+xywin);
    ptlist = [win1 win2];
elseif((idx_ptMin_prev+xywin)>npts)
    % Window overlaps at upper end: take points from lower end
    win2 = (idx_ptMin_prev-xywin):1:npts;
    win1 = 1:(idx_ptMin_prev+xywin-npts);
    ptlist = [win1 win2];
else
    % No overlap: use window
    ptlist = (idx_ptMin_prev-xywin):1:(idx_ptMin_prev+xywin);
end

% Find closest supplied trajectory point to current car position
distances = hypot(p(1) - posx,p(2) - posy);
distances_srch = distances(ptlist);
[ld_ptMin, idx_ptlist] = min(distances_srch);
idx_ptMin = ptlist(idx_ptlist);

% Identify points ahead or behind closest supplied point
if(idx_ptMin == npts)
    % If end of trajectory
    idx_ptFwd = 1;
    idx_ptRev = idx_ptMin-1;
elseif(idx_ptMin == 1)
    % If start of trajectory
    idx_ptFwd = idx_ptMin+1;
    idx_ptRev = npts;
else
    % Standard case
    idx_ptFwd = idx_ptMin+1;
    idx_ptRev = idx_ptMin-1;
end

% Determine if the second point of interest is ahead or behind
ld_ptFwd = distances(idx_ptFwd);
ld_ptRev = distances(idx_ptRev);
if(ld_ptFwd<ld_ptRev)
    idx_a = idx_ptRev;      % CHANGED FROM idx_ptMin
    idx_b = idx_ptFwd;
    dist2fwdpt = ld_ptFwd;
else
    idx_a = idx_ptRev;
    idx_b = idx_ptFwd;     % CHANGED FROM idx_ptMin
    dist2fwdpt = ld_ptFwd; % CHANGED FROM ld_ptFwd
end


% Obtain xy locations for two points of interest
pt_a = [posx(idx_a); posy(idx_a)];
pt_b = [posx(idx_b); posy(idx_b)];

% Find angle between vehicle location, forward point, and track trajectory
vec_b2v  = p(1:2)- pt_b;
vec_b2a  = pt_a  - pt_b;

% Use cosine formula to obtain angle
cos_ang = dot(vec_b2v,vec_b2a)/(norm(vec_b2v)*norm(vec_b2a));

cos_ang = max(cos_ang,eps);
cos_ang = min(cos_ang,1-eps);

% Use angle to obtain lateral distance of vehicle from trajectory
% ld = dist2fwdpt*sin(acos(cos_ang));

% Calculate actual distance including interpolated estimate
ad = dist(idx_b) - dist2fwdpt*cos_ang;

% % Pose targets for Stanley controller (distance cumulatively sums)
dist4interp = [-dist(end)+dist(1:end-1); dist; dist(end)+dist(2:end)];
% posx4interp = [           posx(1:end-1); posx;           posx(2:end)];
% posy4interp = [           posy(1:end-1); posy;           posy(2:end)];
% posz4interp = [           posz(1:end-1); posz;           posz(2:end)];
speed4interp= [          speed(1:end-1);speed;          speed(2:end)];
% 
% % Wrap the interpolation vector for yaw.  
% % Necessary to avoid obtaining values between yaw(end) and yaw(1)
yaw4interp  = [-(yaw(end)-yaw(1)) + yaw(1:end-1);  yaw;  (yaw(end)-yaw(1))+ yaw(2:end)];
% 
% % Current point
% cp = [p(1);p(2);q(3)*180/pi]';
% 
% % Reference point obtained from supplied trajectory
% % Interpolate using Actual distance (ad) + preview distance (pd)
% %----------------------------------------------------------------
% % Increase pd and obtain next point in MPC ref
% 
% %----------------------------------------------------------------
% ref_x    = interp1(dist4interp,posx4interp,ad+pd);
% ref_y    = interp1(dist4interp,posy4interp,ad+pd);
ref_ayaw = interp1(dist4interp,yaw4interp, ad+pd);
% 
% % For visualization only
% ref_z    = interp1(dist4interp,posz4interp,ad+pd);
% 
% 
% % Reference velocity obtained from supplied trajectory
% % Interpolate using actual distance
vx_cp = interp1(dist4interp,speed4interp,ad);
% 
% % Protect for NaNs
% ref_x(isnan(ref_x)) = 0;
% ref_y(isnan(ref_y)) = 0;
ref_ayaw(isnan(ref_ayaw)) = 0;
% ref_z(isnan(ref_z)) = 0;
% 
% Unwrap if necessary after interpolation
if((ad+pd)>dist(end))
   ref_ayaw = ref_ayaw-(yaw(end)-yaw(1));
elseif((ad+pd)<dist(1))
   ref_ayaw = ref_ayaw+(yaw(end)-yaw(1));
end
% 
% % Scale speed target
% % Reduce speed target if car is far from the target trajectory
% % if ld < maxld
    vTarget = vx_cp * speedGain;
% % else
% %     vTarget = minSpd;
% % end
% % vTarget = 10;
% % vTarget = 5;
% % plot(mpc_ref(1,:),mpc_ref(2,:)); hold on
% % Outputs for debugging calculation
% simres = [idx_ptRev idx_ptMin idx_ptFwd ld_ptRev ld_ptMin ld_ptFwd idx_a idx_b ld ad dist2fwdpt cos_ang];
